simulink model "pidControlledUnicycleAndDiffDrive"  (R2016a)
settings: Solver=VariableStepAuto  StartTime=0.0  StopTime=10.0  RelTol=1e-3
libraries: simulink x1
settings Model: Creator=jagni  LastModifiedBy=jagni
settings GRTTargetCC: GeneratePreprocessorConditionals=Use local settings

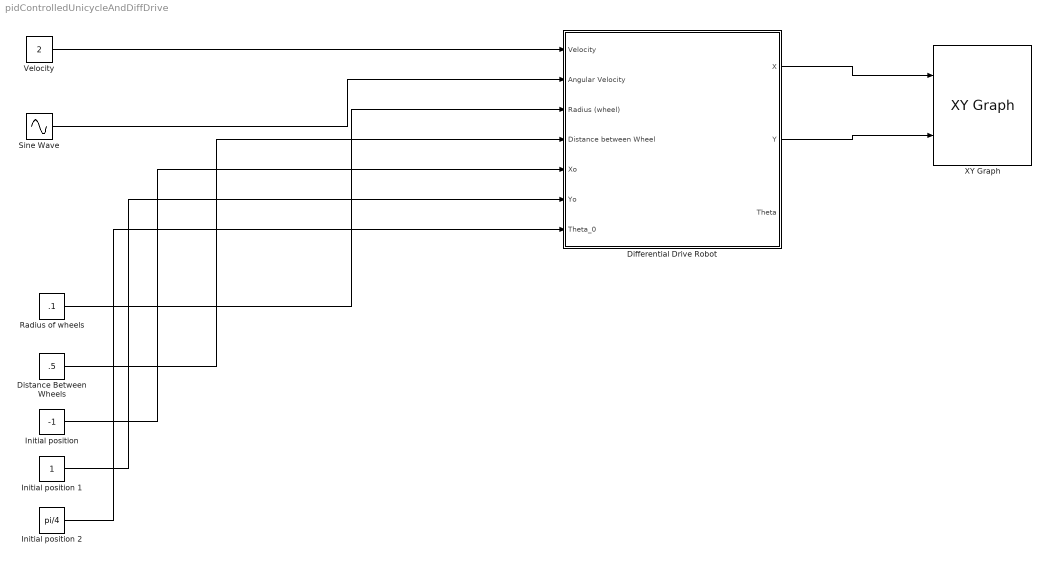
== system pidControlledUnicycleAndDiffDrive ==
  "Differential Drive Robot " : Subsystem
  "Distance Between Wheels " : Constant  Value=.5
  "Initial position " : Constant  Value=-1
  Initial position 1 : Constant
  Initial position 2 : Constant  Value=pi/4
  "Radius of wheels " : Constant  Value=.1
  Sine Wave : Sin  Frequency=.1  SampleTime=0
  "Velocity " : Constant  Value=2
  XY Graph : simulink/Sinks/XY Graph  xmin=-5  xmax=5  ymin=-5  ymax=5  st=1
  wires:
  "Velocity "/1 -> "Differential Drive Robot "/1(Velocity)
  Sine Wave/1 -> "Differential Drive Robot "/2(Angular Velocity)
  "Radius of wheels "/1 -> "Differential Drive Robot "/3(Radius (wheel))
  "Distance Between Wheels "/1 -> "Differential Drive Robot "/4(Distance between Wheel)
  "Differential Drive Robot "/2(Y) -> XY Graph/2
  "Differential Drive Robot "/1(X) -> XY Graph/1
  "Initial position "/1 -> "Differential Drive Robot "/5("Xo ")
  Initial position 1/1 -> "Differential Drive Robot "/6("Yo ")
  Initial position 2/1 -> "Differential Drive Robot "/7(Theta_0)

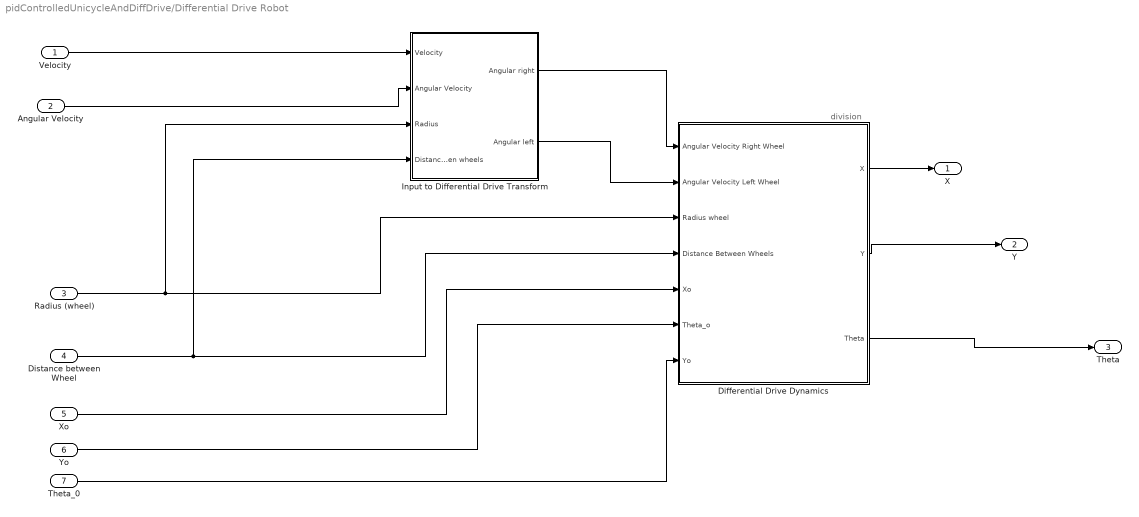
== system pidControlledUnicycleAndDiffDrive/Differential Drive Robot  ==
  note: division
  Velocity : Inport
  Angular Velocity : Inport  Port=2
  Radius (wheel) : Inport  Port=3
  Distance between Wheel : Inport  Port=4
  "Xo " : Inport  Port=5
  "Yo " : Inport  Port=6
  Theta_0 : Inport  Port=7
  "Differential Drive Dynamics " : Subsystem
  "Input to Differential Drive Transform " : Subsystem
  X : Outport
  Y : Outport  Port=2
  "Theta " : Outport  Port=3
  wires:
  Distance between Wheel/1 -> "Input to Differential Drive Transform "/4(Distance between wheels), "Differential Drive Dynamics "/4(Distance Between Wheels)
  "Differential Drive Dynamics "/1(X) -> X/1
  Radius (wheel)/1 -> "Differential Drive Dynamics "/3(Radius wheel), "Input to Differential Drive Transform "/3(Radius)
  "Input to Differential Drive Transform "/1(Angular right) -> "Differential Drive Dynamics "/1(Angular Velocity Right Wheel)
  Velocity/1 -> "Input to Differential Drive Transform "/1(Velocity)
  "Differential Drive Dynamics "/3(Theta) -> "Theta "/1
  "Differential Drive Dynamics "/2(Y) -> Y/1
  "Input to Differential Drive Transform "/2("Angular left ") -> "Differential Drive Dynamics "/2(Angular Velocity Left Wheel)
  Angular Velocity/1 -> "Input to Differential Drive Transform "/2("Angular Velocity ")
  "Xo "/1 -> "Differential Drive Dynamics "/5(Xo)
  "Yo "/1 -> "Differential Drive Dynamics "/6(Theta_o)
  Theta_0/1 -> "Differential Drive Dynamics "/7(Yo)

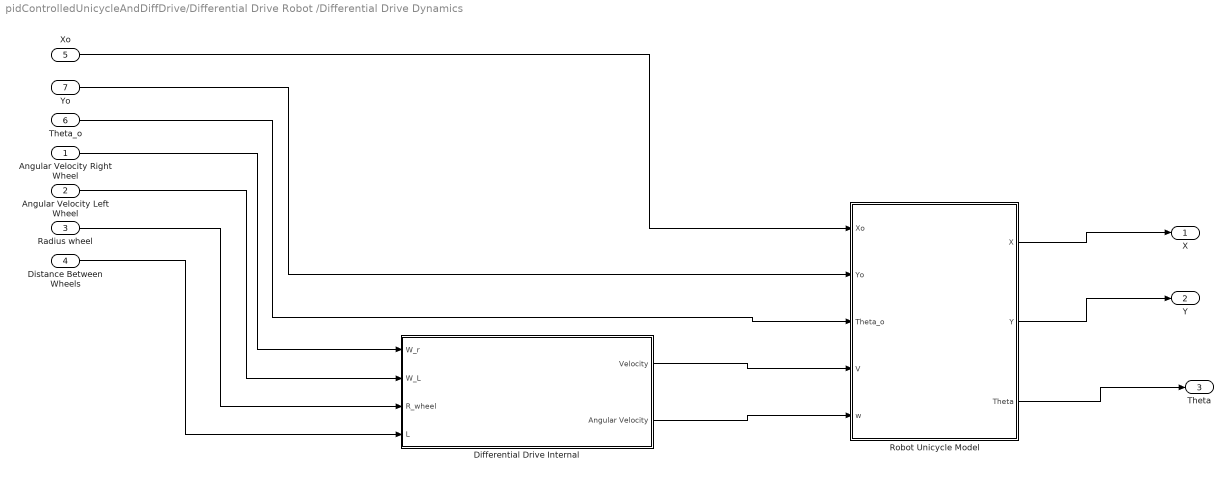
== system pidControlledUnicycleAndDiffDrive/Differential Drive Robot /Differential Drive Dynamics  ==
  Angular Velocity Right Wheel : Inport
  Angular Velocity Left Wheel : Inport  Port=2
  Radius wheel : Inport  Port=3
  Distance Between Wheels : Inport  Port=4
  Xo : Inport  Port=5
  Theta_o : Inport  Port=6
  Yo : Inport  Port=7
  "Differential Drive Internal " : Subsystem
  "Robot Unicycle Model " : Subsystem
  X : Outport
  Y : Outport  Port=2
  Theta : Outport  Port=3
  wires:
  Angular Velocity Right Wheel/1 -> "Differential Drive Internal "/1(W_r)
  "Robot Unicycle Model "/3("Theta ") -> Theta/1
  Distance Between Wheels/1 -> "Differential Drive Internal "/4("L ")
  Radius wheel/1 -> "Differential Drive Internal "/3(R_wheel)
  "Differential Drive Internal "/1("Velocity ") -> "Robot Unicycle Model "/4(V)
  "Differential Drive Internal "/2("Angular Velocity ") -> "Robot Unicycle Model "/5(w)
  "Robot Unicycle Model "/2(Y) -> Y/1
  "Robot Unicycle Model "/1(X) -> X/1
  Angular Velocity Left Wheel/1 -> "Differential Drive Internal "/2(W_L)
  Xo/1 -> "Robot Unicycle Model "/1(Xo)
  Yo/1 -> "Robot Unicycle Model "/2(Yo)
  Theta_o/1 -> "Robot Unicycle Model "/3(Theta_o)

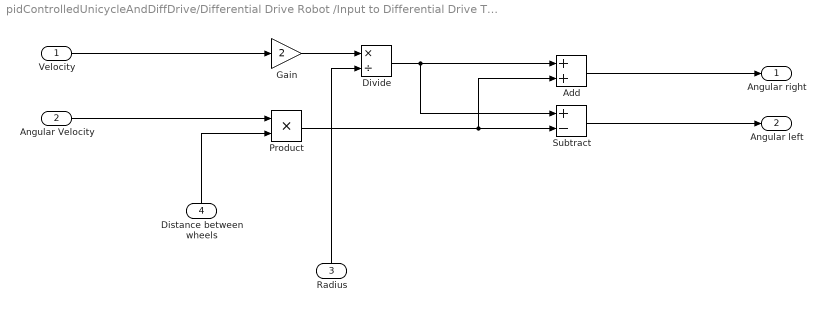
== system pidControlledUnicycleAndDiffDrive/Differential Drive Robot /Input to Differential Drive Transform  ==
  Velocity : Inport
  "Angular Velocity " : Inport  Port=2
  Radius : Inport  Port=3
  Distance between wheels : Inport  Port=4
  Add : Sum
  Divide : Product  Inputs=*/
  Gain : Gain  Gain=2
  Product : Product
  Subtract : Sum  Inputs=+-
  Angular right : Outport
  "Angular left " : Outport  Port=2
  wires:
  Divide/1 -> Add/1, Subtract/1
  "Angular Velocity "/1 -> Product/1
  Product/1 -> Add/2, Subtract/2
  Velocity/1 -> Gain/1
  Gain/1 -> Divide/1
  Distance between wheels/1 -> Product/2
  Radius/1 -> Divide/2
  Add/1 -> Angular right/1
  Subtract/1 -> "Angular left "/1

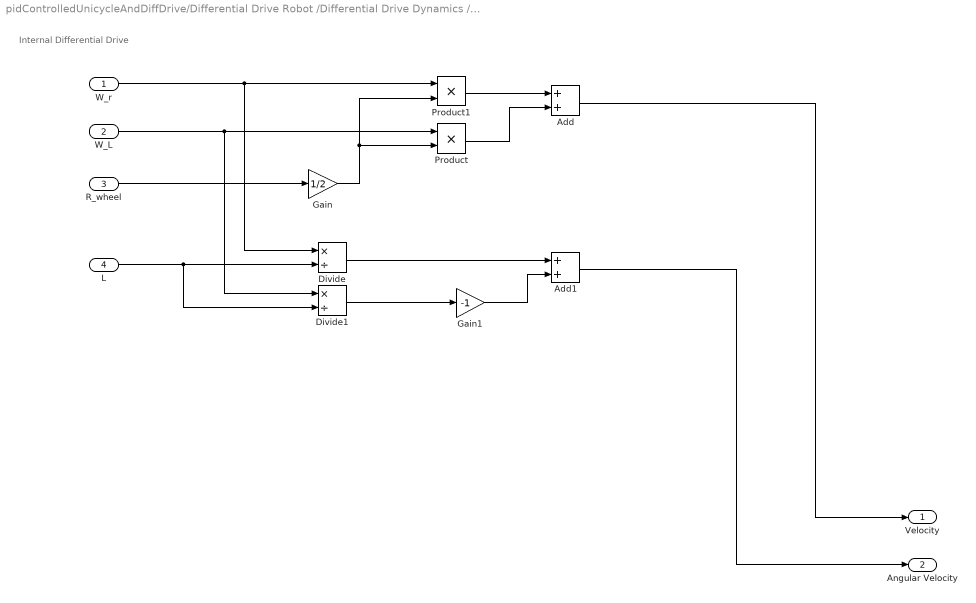
== system pidControlledUnicycleAndDiffDrive/Differential Drive Robot /Differential Drive Dynamics /Differential Drive Internal  ==
  note: Internal Differential Drive
  W_r : Inport
  W_L : Inport  Port=2
  R_wheel : Inport  Port=3
  "L " : Inport  Port=4
  Add : Sum
  Add1 : Sum
  Divide : Product  Inputs=*/
  Divide1 : Product  Inputs=*/
  Gain : Gain  Gain=1/2
  Gain1 : Gain  Gain=-1
  Product : Product
  Product1 : Product
  "Velocity " : Outport
  "Angular Velocity " : Outport  Port=2
  wires:
  Gain/1 -> Product1/2, Product/2
  Product1/1 -> Add/1
  Divide/1 -> Add1/1
  Add/1 -> "Velocity "/1
  Add1/1 -> "Angular Velocity "/1
  Product/1 -> Add/2
  Gain1/1 -> Add1/2
  W_r/1 -> Divide/1, Product1/1
  R_wheel/1 -> Gain/1
  W_L/1 -> Divide1/1, Product/1
  Divide1/1 -> Gain1/1
  "L "/1 -> Divide1/2, Divide/2

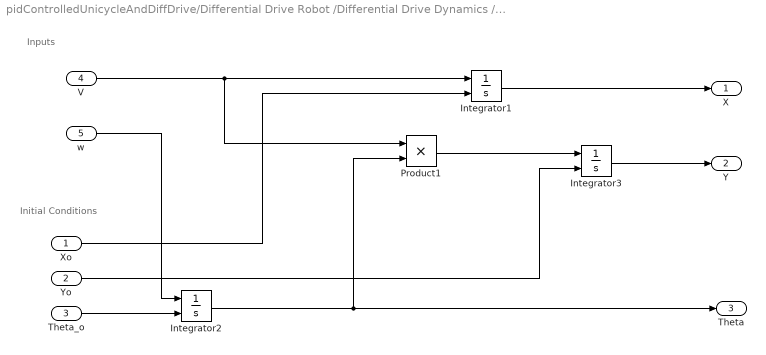
== system pidControlledUnicycleAndDiffDrive/Differential Drive Robot /Differential Drive Dynamics /Robot Unicycle Model  ==
  note: Inputs
  note: Initial Conditions
  Xo : Inport
  Yo : Inport  Port=2
  Theta_o : Inport  Port=3
  V : Inport  Port=4
  w : Inport  Port=5
  Integrator1 : Integrator  InitialConditionSource=external
  Integrator2 : Integrator  InitialConditionSource=external
  Integrator3 : Integrator  InitialConditionSource=external
  Product1 : Product
  X : Outport
  Y : Outport  Port=2
  "Theta " : Outport  Port=3
  wires:
  Theta_o/1 -> Integrator2/2
  w/1 -> Integrator2/1
  V/1 -> Integrator1/1, Product1/1
  Integrator2/1 -> Product1/2, "Theta "/1
  Xo/1 -> Integrator1/2
  Integrator1/1 -> X/1
  Product1/1 -> Integrator3/1
  Integrator3/1 -> Y/1
  Yo/1 -> Integrator3/2
